simulink model "doc_fixpt_vitsoftdec"  (R2014a)
settings: Solver=FixedStepDiscrete  SolverMode=SingleTasking  StartTime=0.0  StopTime=inf  RelTol=1e-3
PreLoadFcn:
  | maxNumErrs = 100;
  | maxNumBits = 1e6;
  | EbNo = 4;
InitFcn:
  | ;
StartFcn:
  | ;
StopFcn:
  | ;
undefined symbols (not defined in the file or in its folder): commblksprivate, Info
libraries: commdigbbndpm3 x2, commcnvcod2 x2, dspquant2 x1, commchan3 x1, commrandsrc2 x1, commsink2 x1
PreSaveFcn:
  | ;
CloseFcn:
  | ;
settings Model: MinMaxOverflowLogging=MinMaxAndOverflow  Creator=The MathWorks Inc.
settings DataIOCC: SignalLoggingSaveFormat=ModelDataLogs  SignalLogging=off  SaveTime=off
settings OptimizationCC: InlineParams=on  ExpressionDepthLimit=2147483647  LocalBlockOutputs=off  InitFltsAndDblsToZero=on  OptimizeModelRefInitCode=on  LifeSpan=1
settings DebuggingCC: SaveWithParameterizedLinksMsg=none  UnderspecifiedInitializationDetection=Classic  SignalResolutionControl=TryResolveAllWithWarning  MultiTaskDSMMsg=warning  MultiTaskCondExecSysMsg=none  FcnCallInpInsideContextMsg=UseLocalSettings  StateNameClashWarn=warning  StrictBusMsg=Warning
settings HardwareCC: ProdBitPerInt=16  ProdIntDivRoundTo=Floor  ProdEndianess=LittleEndian  ProdWordSize=16  ProdHWDeviceType=16-bit Generic  TargetBitPerLong=64  TargetBitPerPointer=64  TargetLongLongMode=on  TargetEndianess=LittleEndian  TargetWordSize=64  TargetHWDeviceType=MATLAB Host  ProdEqTarget=off
settings RTWCC: SystemTargetFile=ert.tlc  TemplateMakefile=ert_default_tmf  Description=Real-Time Workshop Embedded Coder (no auto configuration)  GenerateReport=on  RetainRTWFile=on  ProcessScript=ert_make_rtw_hook  IncludeHyperlinkInReport=on  LaunchReport=on  IncludeERTFirstTime=on
settings CodeAppCC: CustomSymbolStrType=$N$R$M  InternalIdentifier=Classic
settings ERTTargetCC: TargetFcnLib=ansi_tfl_tmw.mat  ParMdlRefBuildCompliant=on  CompOptLevelCompliant=on  ConcurrentExecutionCompliant=on  ERTFirstTimeCompliant=on  SupportAbsoluteTime=off  MatFileLogging=on  ModelStepFunctionPrototypeControlCompliant=on  CPPClassGenCompliant=on  ERTCustomFileTemplate=example_file_process.tlc

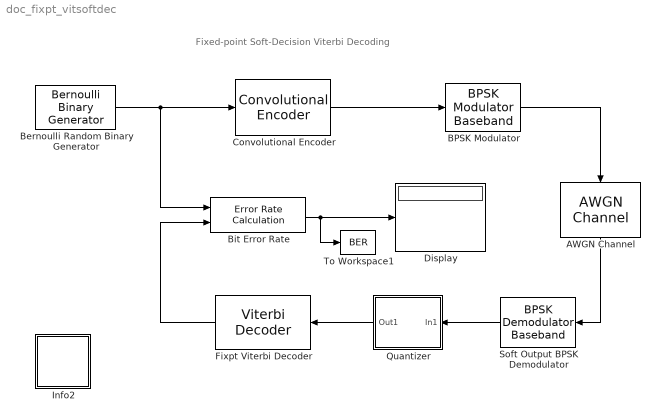
== system doc_fixpt_vitsoftdec ==
  note: Fixed-point Soft-Decision Viterbi Decoding
  " Quantizer" : Subsystem
  AWGN Channel : commchan3/AWGN Channel  InputProcessing=Columns as channels (frame based)  seed=113  noiseMode="Signal to noise ratio  (Eb/No)"  EbNodB=EbNo - 10*log10(2)  EsNodB=1  SNRdB=10  bitsPerSym=1  Ps=1  Tsym=0.005  variance=(1*0.005)/((1/200)*10^(EbNo/10))
  BPSK Modulator : commdigbbndpm3/BPSK Modulator Baseband  Ph=0  outDtype=double  outWordLen=16  outUDDataType=sfix(16)  outFracLenMode=Best precision  outFracLen=15
  Bernoulli Random Binary Generator : commrandsrc2/Bernoulli Binary Generator  P=0.5  seed=911  Ts=0.01  frameBased=on  sampPerFrame=100  orient=off  outDataType=boolean
  Bit Error Rate : commsink2/Error Rate Calculation  N=56  st_delay=0  cp_mode=Entire frame  subframe=[]  PMode=Port  WsName=ErrorVec  RsMode2=off  stop=on  numErr=maxNumErrs  maxBits=maxNumBits
  Convolutional Encoder : commcnvcod2/Convolutional Encoder  trellis=poly2trellis(9, [561 753])  opMode=Continuous  DelayedResetAction=off  hasIniStPort=off  hasFinStPort=off  usePuncVector=off  punctureVector=[1 1 0 1 1 0].'  reset=Unused parameter value
  Display : Display
  Fixpt Viterbi Decoder : commcnvcod2/Viterbi Decoder  trellis=poly2trellis(9, [561 753])  isPunctured=off  punctureVector=[1 1 0 1 1 0].'  erasures=off  dectype=Soft decision  runSigValErrCheck=off  nsdecb=3  smWordLength=6  tbdepth=56  opmode=Continuous  reset=off  outDataType=boolean  delayedResetAction=off
  Info2 : Subsystem  AncestorBlock=commblksprivate/Info  mask(Info){}
      settings: OpenFcn=helpview([docroot '/toolbox/comm/comm.map'], 'doc_fixpt_vitsoftdec')
      mask Display: disp('Info')
  Soft Output BPSK Demodulator : commdigbbndpm3/BPSK Demodulator Baseband  Ph=0  DecType=Log-likelihood ratio  VarSource=Dialog  Variance=1/(10^((EbNo-10*log10(2))/10))  outDtype=double  derotateFactorWordLen=16
  To Workspace1 : ToWorkspace  VariableName=BER  SampleTime=-1
      settings: MaxDataPoints=1
  wires:
  Bernoulli Random Binary Generator/1 -> Convolutional Encoder/1, Bit Error Rate/1
  Convolutional Encoder/1 -> BPSK Modulator/1
  AWGN Channel/1 -> Soft Output BPSK Demodulator/1
  BPSK Modulator/1 -> AWGN Channel/1
  Bit Error Rate/1 -> To Workspace1/1, Display/1
  Fixpt Viterbi Decoder/1 -> Bit Error Rate/2
  Soft Output BPSK Demodulator/1 -> " Quantizer"/1(In1)
  " Quantizer"/1(Out1) -> Fixpt Viterbi Decoder/1

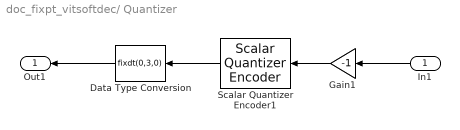
== system doc_fixpt_vitsoftdec/ Quantizer ==
  In1 : Inport
  Data Type Conversion : DataTypeConversion  OutDataTypeStr=fixdt(0,3,0)
  Gain1 : Gain  Gain=-1
  Scalar Quantizer Encoder1 : dspquant2/Scalar Quantizer Encoder  paramSrc=Specify via dialog  partType=Unbounded  BBoundary=[-6:2:6]/4  UBoundary=[-3:3]  SearchMethod=Linear  tieBreakRule=Choose the higher index  outQU=off  outQError=off  codebook=[1.5:9.5]  outStatus=off  invalidin=Clip  idtype=uint8  roundingMode=Floor  overflowMode=off
  Out1 : Outport
  wires:
  In1/1 -> Gain1/1
  Data Type Conversion/1 -> Out1/1
  Scalar Quantizer Encoder1/1 -> Data Type Conversion/1
  Gain1/1 -> Scalar Quantizer Encoder1/1

== system doc_fixpt_vitsoftdec/Info2 ==
